simulink model "mrac"  (R2018a)
settings: Solver=VariableStepAuto  StartTime=0.0  StopTime=50.0  MaxStep=1e-1  RelTol=1e-3
settings Model: Creator=saad  LastModifiedBy=saad

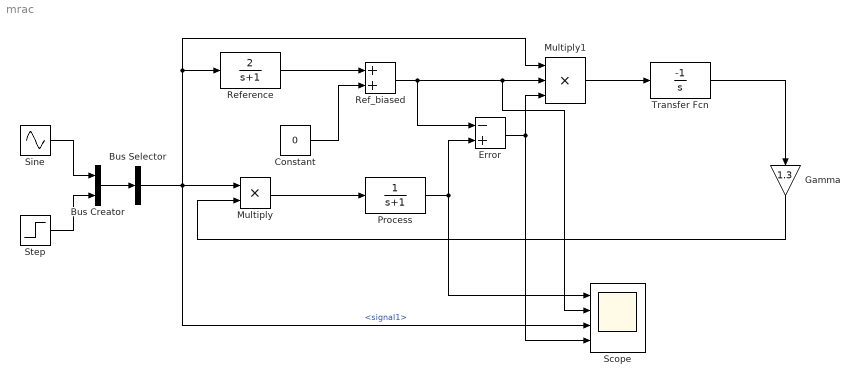
== system mrac ==
  Bus Selector : BusSelector  OutputSignals=signal1
  Bus Creator : BusCreator  Inputs=2
  Constant : Constant  Value=0
  Error : Sum  Inputs=-+
  Gamma : Gain  Gain=1.3
  Multiply : Product
  Multiply1 : Product  Inputs=3
  Process : TransferFcn  Denominator=[1 1]
  Ref_biased : Sum
  Reference : TransferFcn  Numerator=[2]  Denominator=[1 1]
  Scope : Scope  NumInputPorts=4
  Sine : Sin  SampleTime=0
  "Step " : Step  SampleTime=0
  Transfer Fcn : TransferFcn  Numerator=[-1]  Denominator=[1 0]
  wires:
  Multiply/1 -> Process/1
  Multiply1/1 -> Transfer Fcn/1
  Process/1 -> Scope/1, Error/2
  Error/1 -> Scope/4, Multiply1/3
  Sine/1 -> Bus Creator/1
  "Step "/1 -> Bus Creator/2
  Bus Creator/1 -> Bus Selector/1
  Bus Selector/1 -> Scope/3, Reference/1, Multiply1/1, Multiply/1  "<signal1>"
  Transfer Fcn/1 -> Gamma/1
  Gamma/1 -> Multiply/2
  Ref_biased/1 -> Error/1, Scope/2, Multiply1/2
  Reference/1 -> Ref_biased/1
  Constant/1 -> Ref_biased/2
